simulink model "c7mdde6"  (Simulink 7.7)
settings: Solver=ode45  StartTime=0.0  StopTime=80.0  RelTol=1e-8
settings Model: Creator=Administrator  LastModifiedBy=Professor Dingyu Xue
settings DataIOCC: LimitDataPoints=off
settings OptimizationCC: InitFltsAndDblsToZero=on
settings DebuggingCC: StrictBusMsg=Warning
settings CodeAppCC: CustomSymbolStrType=$N$R$M_T
settings GRTTargetCC: TargetFunctionLibrary=NOT IN USE  CPPClassGenCompliant=on

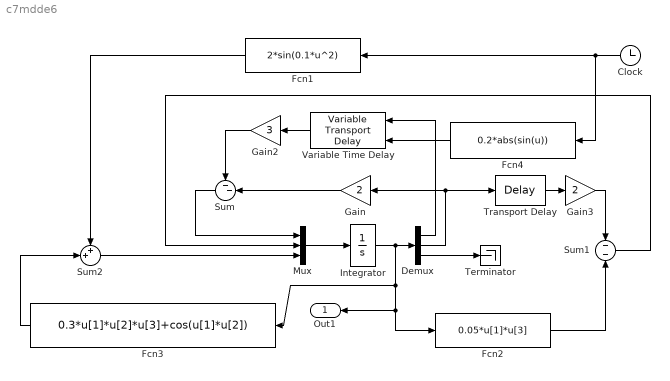
== system c7mdde6 ==
  Clock : Clock
      settings: Decimation=10
  Demux : Demux  Outputs=3
  Fcn1 : Fcn  Expr=2*sin(0.1*u^2)
  Fcn2 : Fcn  Expr=0.05*u[1]*u[3]
  Fcn3 : Fcn  Expr=0.3*u[1]*u[2]*u[3]+cos(u[1]*u[2])
  Fcn4 : Fcn  Expr=0.2*abs(sin(u))
  Gain : Gain  Gain=2
  Gain2 : Gain  Gain=3
  Gain3 : Gain  Gain=2
  Integrator : Integrator  InitialCondition=[1; 1; 1]
  Mux : Mux  Inputs=3
  Sum : Sum  Inputs=--|
  Sum1 : Sum  Inputs=-|-
  Sum2 : Sum  Inputs=++|
  Terminator : Terminator
  Transport Delay : TransportDelay  DelayTime=0.8
  Variable Time Delay : VariableTransportDelay  MaximumDelay=10
  Out1 : Outport
  wires:
  Mux/1 -> Integrator/1
  Integrator/1 -> Demux/1, Fcn3/1, Fcn2/1, Out1/1
  Demux/3 -> Terminator/1
  Demux/2 -> Gain/1, Transport Delay/1
  Sum/1 -> Mux/1
  Gain/1 -> Sum/2
  Demux/1 -> Variable Time Delay/1
  Clock/1 -> Fcn1/1, Fcn4/1
  Variable Time Delay/1 -> Gain2/1
  Gain2/1 -> Sum/1
  Transport Delay/1 -> Gain3/1
  Fcn2/1 -> Sum1/2
  Sum2/1 -> Mux/3
  Fcn3/1 -> Sum2/2
  Fcn1/1 -> Sum2/1
  Sum1/1 -> Mux/2
  Gain3/1 -> Sum1/1
  Fcn4/1 -> Variable Time Delay/2
